simulink model "CTF"  (R2015a)
settings: Solver=ode15s  StartTime=0.0  StopTime=1e5  MaxStep=50  RelTol=1e-3
libraries: simCryogenics_lib x74, nesl_utility x45
settings Model: Creator=GM246266  LastModifiedBy=FB229602
settings SimscapeCC: SimscapeLogType=all

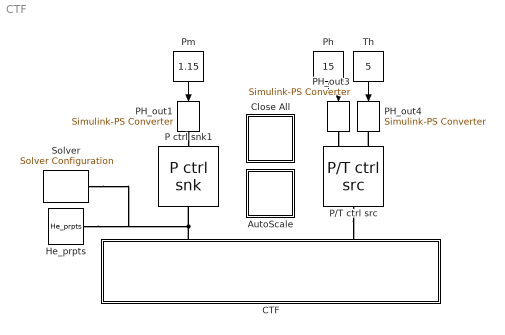
== system CTF ==
  AutoScale : Subsystem
      settings: OpenFcn=|
      | set(0, 'showhiddenhandles', 'on')
      | 
      | scope = findobj(0, 'Tag', 'SIMULINK_SIMSCOPE_FIGURE');
      | 
      | for i=1:length(scope)
      |   simscope('ScopeBar', 'ActionIcon', 'Find',     scope(i))
      | end
      | 
      | set(0, 'showhiddenhandles', 'off')
      mask Display: disp('Auto\nScale\nScope')
  CTF : Subsystem
  Close All : Subsystem
      settings: OpenFcn=|
      | set(0, 'showhiddenhandles', 'on')
      | scope = findobj(0, 'Tag','SIMULINK_SIMSCOPE_FIGURE');
      | close(scope)
      | set(0, 'showhiddenhandles', 'off')
      mask Display: disp('Close\nAll\nScope')
  He_prpts : simCryogenics_lib/Utilities/He_prpts  P_min=0.1 bar  T_min=3 K  T_max=8 K  P_max=20 bar  Mol=4.0026 * 10 ^ (- 3) kg/mol
  P ctrl snk1 : simCryogenics_lib/Sources_Sinks/P ctrl snk
  P/T ctrl src : simCryogenics_lib/Sources_Sinks/P//T ctrl src
  PH_out1 : nesl_utility/Simulink-PS Converter  PhysicalDomain=network_engine_domain  SubClassName=ps_input  LeftPortType=input  RightPortType=output  PseudoPeriodic=off  Frequencies=[]  NoiseDistribution=none  NoiseParameters=[]  Unit=bar  AffineConversion=off  InputFiltering=off  SimscapeFilterOrder=1  InputFilterTimeConstant=0.001  UdotUserProvided=1
  PH_out3 : nesl_utility/Simulink-PS Converter  PhysicalDomain=network_engine_domain  SubClassName=ps_input  LeftPortType=input  RightPortType=output  PseudoPeriodic=off  Frequencies=[]  NoiseDistribution=none  NoiseParameters=[]  Unit=bar  AffineConversion=off  InputFiltering=off  SimscapeFilterOrder=1  InputFilterTimeConstant=0.001  UdotUserProvided=1
  PH_out4 : nesl_utility/Simulink-PS Converter  PhysicalDomain=network_engine_domain  SubClassName=ps_input  LeftPortType=input  RightPortType=output  PseudoPeriodic=off  Frequencies=[]  NoiseDistribution=none  NoiseParameters=[]  Unit=K  AffineConversion=off  InputFiltering=off  SimscapeFilterOrder=1  InputFilterTimeConstant=0.001  UdotUserProvided=1
  Ph : Constant  Value=15
  Pm : Constant  Value=1.15
  Solver : nesl_utility/Solver Configuration  PhysicalDomain=network_engine_domain  SubClassName=solver  LeftPortType=input  RightPortType=generic  Accelerate=off  Tones=[]  Harmonics=[]  SimulateNoise=off  Profile=off  UseLocalSampling=off  EnableSwitchedLinearOptims=on  FrequencyDomain=off  UseCCode=off  RelTol=0.001  AbsTol=1e-06  MinStep=1e-09  ToWorkspace=off  RevertToSquareIcSolve=off  NumHomotopyIterations=100  DoDC=off  ResidualTolerance=1e-09  UseLocalSolver=off  LocalSolverChoice=NE_BACKWARD_EULER_ADVANCER  LocalSolverSampleTime=0.001  DoFixedCost=off  MaxNonlinIter=3  MaxModeIter=2  LinearAlgebra=Sparse  DelaysMemoryBudget=1024  AutomaticFiltering=on  FilteringTimeConstant=0.001
  Th : Constant  Value=5
  wires:
  Th/1 -> PH_out4/1
  Ph/1 -> PH_out3/1
  Pm/1 -> PH_out1/1
  connections:
  PH_out1/RConn1 -- P ctrl snk1/LConn1
  PH_out3/RConn1 -- P/T ctrl src/LConn1
  P/T ctrl src/LConn2 -- PH_out4/RConn1
  CTF/RConn1 -- Solver/RConn1 -- He_prpts/RConn1 -- P ctrl snk1/RConn1
  P/T ctrl src/RConn1 -- CTF/RConn2

== system CTF/AutoScale ==

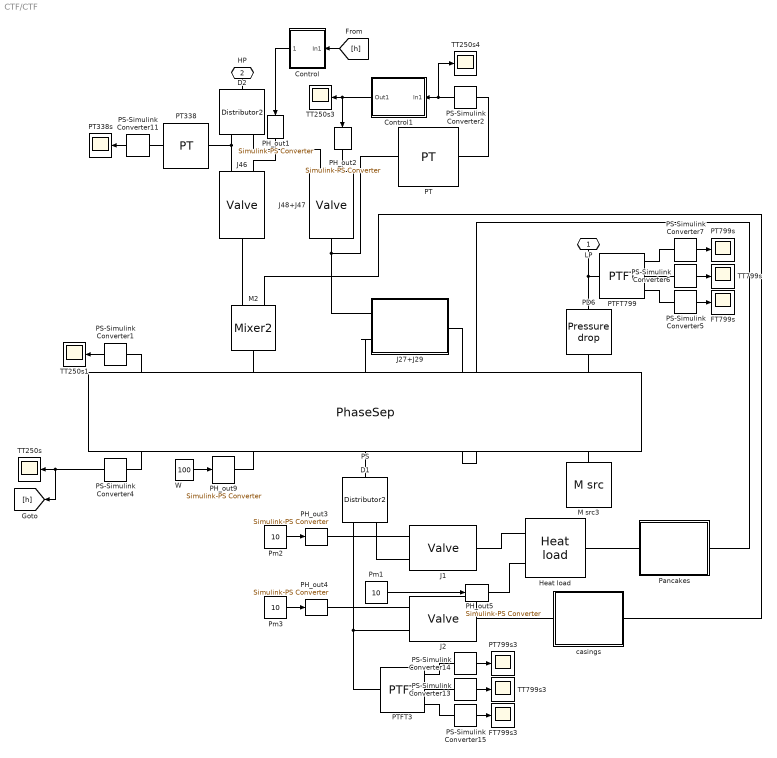
== system CTF/CTF ==
  Control : Subsystem
  Control1 : Subsystem
  D1 : simCryogenics_lib/Elements/Distributor2
  D2 : simCryogenics_lib/Elements/Distributor2
  FT799s : Scope
      settings: SaveName=FT799
  FT799s3 : Scope
      settings: SaveName=FT2
  Heat load : simCryogenics_lib/Utilities/Heat load
  J1 : simCryogenics_lib/Elements/Valve  CVmax=20  ControlInputMin=0  ControlInputMax=100  Xt=0.86  Rv=10  lin_v=0  lim_v=0  K=2.4e-5 m^1.50000*kg^0.50000/s/bar^0.50000  Cmd_specify=off  Cmd_priority=High  Cmd=0  gamma_specify=off  gamma_priority=High  gamma=0  rho_specify=off  rho_priority=High  rho=0 kg/m^3  Xc_specify=off  Xc_priority=High  Xc=0  X_specify=off  X_priority=High  X=0  Y_specify=off  Y_priority=High  Y=0  CV_specify=off  CV_priority=High  CV=0
  J2 : simCryogenics_lib/Elements/Valve  CVmax=25  ControlInputMin=0  ControlInputMax=100  Xt=0.86  Rv=10  lin_v=0  lim_v=0  K=2.4e-5 m^1.50000*kg^0.50000/s/bar^0.50000  Cmd_specify=off  Cmd_priority=High  Cmd=0  gamma_specify=off  gamma_priority=High  gamma=0  rho_specify=off  rho_priority=High  rho=0 kg/m^3  Xc_specify=off  Xc_priority=High  Xc=0  X_specify=off  X_priority=High  X=0  Y_specify=off  Y_priority=High  Y=0  CV_specify=off  CV_priority=High  CV=0
  J27+J29 : Subsystem
  J46 : simCryogenics_lib/Elements/Valve  CVmax=0.55  ControlInputMin=0  ControlInputMax=100  Xt=0.86  Rv=10  lin_v=0  lim_v=0  K=2.4e-5 m^1.50000*kg^0.50000/s/bar^0.50000  Cmd_specify=off  Cmd_priority=High  Cmd=0  gamma_specify=off  gamma_priority=High  gamma=0  rho_specify=off  rho_priority=High  rho=0 kg/m^3  Xc_specify=off  Xc_priority=High  Xc=0  X_specify=off  X_priority=High  X=0  Y_specify=off  Y_priority=High  Y=0  CV_specify=off  CV_priority=High  CV=0
  J48+J47 : simCryogenics_lib/Elements/Valve  CVmax=0.55  ControlInputMin=0  ControlInputMax=100  Xt=0.86  Rv=10  lin_v=0  lim_v=0  K=2.4e-5 m^1.50000*kg^0.50000/s/bar^0.50000  Cmd_specify=off  Cmd_priority=High  Cmd=0  gamma_specify=off  gamma_priority=High  gamma=0  rho_specify=off  rho_priority=High  rho=0 kg/m^3  Xc_specify=off  Xc_priority=High  Xc=0  X_specify=off  X_priority=High  X=0  Y_specify=off  Y_priority=High  Y=0  CV_specify=off  CV_priority=High  CV=0
  M src3 : simCryogenics_lib/Sources_Sinks/M src  M=0 kg/s
  M2 : simCryogenics_lib/Elements/Mixer2
  PD6 : simCryogenics_lib/Utilities/Pressure drop  K=1 s*bar/kg
  PH_out{1..4} (4 alike) : nesl_utility/Simulink-PS Converter  PhysicalDomain=network_engine_domain  SubClassName=ps_input  LeftPortType=input  RightPortType=output  PseudoPeriodic=off  Frequencies=[]  NoiseDistribution=none  NoiseParameters=[]  Unit=bar  AffineConversion=off  InputFiltering=off  SimscapeFilterOrder=1  InputFilterTimeConstant=0.001  UdotUserProvided=1
  PH_out5 : nesl_utility/Simulink-PS Converter  PhysicalDomain=network_engine_domain  SubClassName=ps_input  LeftPortType=input  RightPortType=output  PseudoPeriodic=off  Frequencies=[]  NoiseDistribution=none  NoiseParameters=[]  Unit=W  AffineConversion=off  InputFiltering=off  SimscapeFilterOrder=1  InputFilterTimeConstant=0.001  UdotUserProvided=1
  PH_out9 : nesl_utility/Simulink-PS Converter  PhysicalDomain=network_engine_domain  SubClassName=ps_input  LeftPortType=input  RightPortType=output  PseudoPeriodic=off  Frequencies=[]  NoiseDistribution=none  NoiseParameters=[]  Unit=1  AffineConversion=off  InputFiltering=off  SimscapeFilterOrder=1  InputFilterTimeConstant=0.001  UdotUserProvided=1
  PS : simCryogenics_lib/Elements/PhaseSep  Ideal1=1  DeltaT1=0.05 K  N1=1  h1=1 W/K  Ideal2=1  DeltaT2=0.05 K  N2=1  h2=1 W/K  hmax=1 m  S=1 m^2  P0=1.089 bar  h0=50
  PS-Simulink Converter{1..2,4..7,11,13..15} (10 alike) : nesl_utility/PS-Simulink Converter  PhysicalDomain=network_engine_domain  SubClassName=ps_output  LeftPortType=input  RightPortType=output  PseudoPeriodic=off  Frequencies=[]  Unit=1  AffineConversion=off
  PT : simCryogenics_lib/Sensors/PT
  PT338 : simCryogenics_lib/Sensors/PT
  PT338s : Scope
      settings: SaveName=PT1
  PT799s : Scope
      settings: SaveName=PT3
  PT799s3 : Scope
      settings: SaveName=PT4
  PTFT3 : simCryogenics_lib/Sensors/PTFT
  PTFT799 : simCryogenics_lib/Sensors/PTFT
  Pancakes : Subsystem
  Pm1 : Constant  Value=10
  Pm2 : Constant  Value=10
  Pm3 : Constant  Value=10
  TT250s{,1,3..4} (4 alike) : Scope
      TT250s settings: TimeRange=100000  YMin=49.99  YMax=50.08000000000001  SaveName=TT
      TT250s1 settings: SaveName=TT1
      TT250s3 settings: TimeRange=100000  YMin=49.99  YMax=50.08000000000001  SaveName=TT6
      TT250s4 settings: TimeRange=100000  YMin=1.8  YMax=3.1  SaveName=TT7
  TT799s : Scope
      settings: SaveName=TT799
  TT799s3 : Scope
      settings: SaveName=TT4
  W : Constant  Value=100
  casings : Subsystem
  LP : PMIOPort  Port=1  Side=Right
  HP : PMIOPort  Port=2  Side=Right
  wires:
  PS-Simulink Converter1/1 -> TT250s1/1
  W/1 -> PH_out9/1
  PS-Simulink Converter11/1 -> PT338s/1
  PS-Simulink Converter7/1 -> PT799s/1
  PS-Simulink Converter5/1 -> FT799s/1
  PS-Simulink Converter6/1 -> TT799s/1
  Control1/1(Out1) -> PH_out2/1, TT250s3/1
  Pm2/1 -> PH_out3/1
  Pm3/1 -> PH_out4/1
  PS-Simulink Converter14/1 -> PT799s3/1
  PS-Simulink Converter15/1 -> FT799s3/1
  PS-Simulink Converter13/1 -> TT799s3/1
  PS-Simulink Converter4/1 -> [h], TT250s/1
  Control/1(Out1) -> PH_out1/1
  PS-Simulink Converter2/1 -> TT250s4/1, Control1/1(In1)
  [h] -> Control/1(In1)
  Pm1/1 -> PH_out5/1
  connections:
  PT338/LConn1 -- J46/LConn2 -- D2/RConn2
  LP/RConn1 -- PD6/RConn1 -- PTFT799/LConn1
  M2/RConn1 -- PS/LConn4
  PS-Simulink Converter7/LConn1 -- PTFT799/RConn1
  PS-Simulink Converter1/LConn1 -- PS/LConn5
  M src3/RConn1 -- PS/RConn1
  PS-Simulink Converter5/LConn1 -- PTFT799/RConn3
  PS-Simulink Converter4/LConn1 -- PS/RConn5
  PS-Simulink Converter6/LConn1 -- PTFT799/RConn2
  PH_out9/RConn1 -- PS/RConn4
  PD6/LConn1 -- PS/LConn1
  PT338/RConn1 -- PS-Simulink Converter11/LConn1
  Pancakes/RConn1 -- PS/LConn2
  J27+J29/LConn2 -- PS/LConn3
  J27+J29/RConn1 -- PS/RConn2
  PT/LConn1 -- J48+J47/RConn1 -- J27+J29/LConn1
  J2/RConn1 -- casings/LConn1
  J46/RConn1 -- M2/LConn2
  D1/LConn1 -- PS/RConn3
  D1/RConn2 -- PTFT3/LConn1 -- J2/LConn2
  PH_out1/RConn1 -- J46/LConn1
  PH_out2/RConn1 -- J48+J47/LConn1
  PH_out3/RConn1 -- J1/LConn1
  J2/LConn1 -- PH_out4/RConn1
  HP/RConn1 -- D2/LConn1
  D2/RConn1 -- J48+J47/LConn2
  PS-Simulink Converter13/LConn1 -- PTFT3/RConn2
  PS-Simulink Converter15/LConn1 -- PTFT3/RConn3
  PS-Simulink Converter14/LConn1 -- PTFT3/RConn1
  D1/RConn1 -- J1/LConn2
  casings/RConn1 -- M2/LConn1
  PS-Simulink Converter2/LConn1 -- PT/RConn1
  PH_out5/RConn1 -- Heat load/LConn2
  J1/RConn1 -- Heat load/LConn1
  Heat load/RConn1 -- Pancakes/LConn1

== system CTF/Close All ==

== system CTF/CTF/Control ==
  In1 : Inport
  Bias : Bias  Bias=+60
  Gain : Gain  Gain=-1
  Out1 : Outport
  wires:
  Bias/1 -> Out1/1
  Gain/1 -> Bias/1
  In1/1 -> Gain/1

== system CTF/CTF/Control1 ==
  In1 : Inport
  Bias : Bias  Bias=-3
  Bias1 : Bias  Bias=10
  Gain : Gain  Gain=-10
  Out1 : Outport
  wires:
  Bias/1 -> Gain/1
  In1/1 -> Bias/1
  Gain/1 -> Bias1/1
  Bias1/1 -> Out1/1

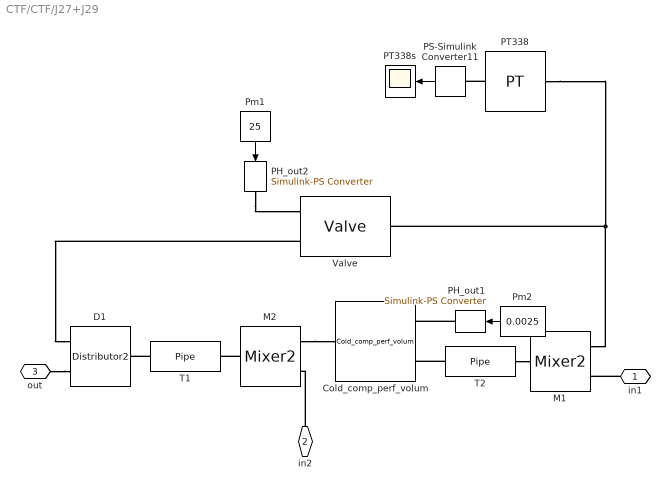
== system CTF/CTF/J27+J29 ==
  Cold_comp_perf_volum : simCryogenics_lib/Elements/Cold_comp_perf_volum  P0=1 bar  eta=0.8  Sin_specify=off  Sin_priority=High  Sin=0 kJ/kg  HoutIs_specify=off  HoutIs_priority=High  HoutIs=0 kJ/kg
  D1 : simCryogenics_lib/Elements/Distributor2
  M1 : simCryogenics_lib/Elements/Mixer2
  M2 : simCryogenics_lib/Elements/Mixer2
  PH_out1 : nesl_utility/Simulink-PS Converter  PhysicalDomain=network_engine_domain  SubClassName=ps_input  LeftPortType=input  RightPortType=output  PseudoPeriodic=off  Frequencies=[]  NoiseDistribution=none  NoiseParameters=[]  Unit=1  AffineConversion=off  InputFiltering=off  SimscapeFilterOrder=1  InputFilterTimeConstant=0.001  UdotUserProvided=1
  PH_out2 : nesl_utility/Simulink-PS Converter  PhysicalDomain=network_engine_domain  SubClassName=ps_input  LeftPortType=input  RightPortType=output  PseudoPeriodic=off  Frequencies=[]  NoiseDistribution=none  NoiseParameters=[]  Unit=bar  AffineConversion=off  InputFiltering=off  SimscapeFilterOrder=1  InputFilterTimeConstant=0.001  UdotUserProvided=1
  PS-Simulink Converter11 : nesl_utility/PS-Simulink Converter  PhysicalDomain=network_engine_domain  SubClassName=ps_output  LeftPortType=input  RightPortType=output  PseudoPeriodic=off  Frequencies=[]  Unit=1  AffineConversion=off
  PT338 : simCryogenics_lib/Sensors/PT
  PT338s : Scope
      settings: SaveName=PT5
  Pm1 : Constant  Value=25
  Pm2 : Constant  Value=0.0025
  T1 : simCryogenics_lib/Elements/Pipe  Vol=0.01 m^3  Ideal=0  P0=3 bar  T0=5 K
  T2 : simCryogenics_lib/Elements/Pipe  Vol=0.01 m^3  Ideal=0  P0=1 bar  T0=5 K
  Valve : simCryogenics_lib/Elements/Valve  CVmax=0.55  ControlInputMin=0  ControlInputMax=100  Xt=0.86  Rv=10  lin_v=0  lim_v=0  K=2.4e-5 m^1.50000*kg^0.50000/s/bar^0.50000  Cmd_specify=off  Cmd_priority=High  Cmd=0  gamma_specify=off  gamma_priority=High  gamma=0  rho_specify=off  rho_priority=High  rho=0 kg/m^3  Xc_specify=off  Xc_priority=High  Xc=0  X_specify=off  X_priority=High  X=0  Y_specify=off  Y_priority=High  Y=0  CV_specify=off  CV_priority=High  CV=0
  in1 : PMIOPort  Port=1  Side=Right
  in2 : PMIOPort  Port=2  Side=Left
  out : PMIOPort  Port=3  Side=Left
  wires:
  Pm1/1 -> PH_out2/1
  Pm2/1 -> PH_out1/1
  PS-Simulink Converter11/1 -> PT338s/1
  connections:
  T1/RConn1 -- D1/LConn1
  PH_out1/RConn1 -- Cold_comp_perf_volum/LConn2
  PH_out2/RConn1 -- Valve/LConn1
  Valve/LConn2 -- D1/RConn2
  out/RConn1 -- D1/RConn1
  in1/RConn1 -- M1/LConn1
  M1/LConn2 -- PT338/LConn1 -- Valve/RConn1
  T2/RConn1 -- Cold_comp_perf_volum/LConn1
  T2/LConn1 -- M1/RConn1
  M2/RConn1 -- T1/LConn1
  M2/LConn2 -- Cold_comp_perf_volum/RConn1
  in2/RConn1 -- M2/LConn1
  PT338/RConn1 -- PS-Simulink Converter11/LConn1

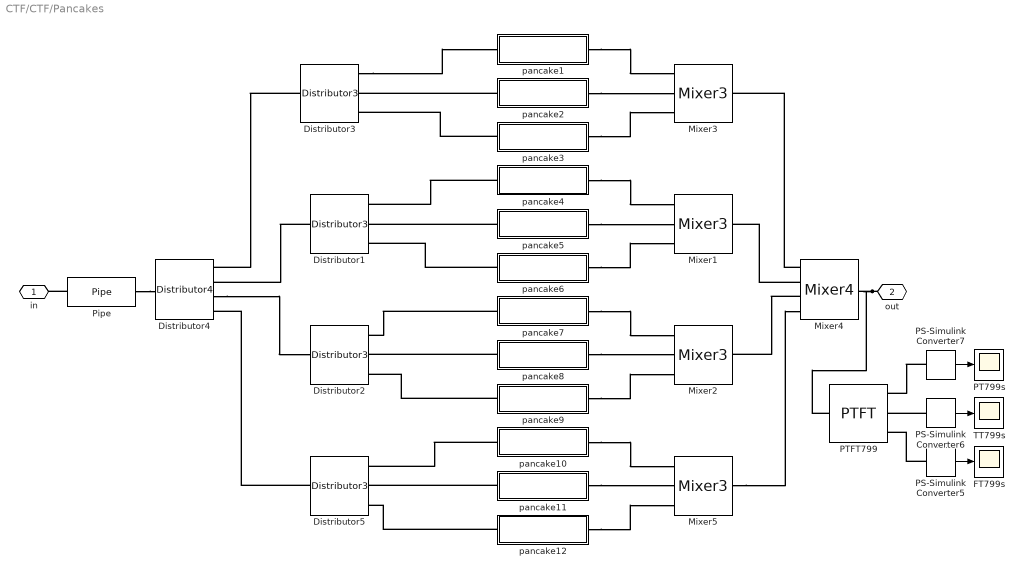
== system CTF/CTF/Pancakes ==
  Distributor{1..3,5} (4 alike) : simCryogenics_lib/Elements/Distributor3
  Distributor4 : simCryogenics_lib/Elements/Distributor4
  FT799s : Scope
      settings: SaveName=FT
  Mixer{1..3,5} (4 alike) : simCryogenics_lib/Elements/Mixer3
  Mixer4 : simCryogenics_lib/Elements/Mixer4
  PS-Simulink Converter5 : nesl_utility/PS-Simulink Converter  PhysicalDomain=network_engine_domain  SubClassName=ps_output  LeftPortType=input  RightPortType=output  PseudoPeriodic=off  Frequencies=[]  Unit=1  AffineConversion=off
  PS-Simulink Converter6 : nesl_utility/PS-Simulink Converter  PhysicalDomain=network_engine_domain  SubClassName=ps_output  LeftPortType=input  RightPortType=output  PseudoPeriodic=off  Frequencies=[]  Unit=1  AffineConversion=off
  PS-Simulink Converter7 : nesl_utility/PS-Simulink Converter  PhysicalDomain=network_engine_domain  SubClassName=ps_output  LeftPortType=input  RightPortType=output  PseudoPeriodic=off  Frequencies=[]  Unit=1  AffineConversion=off
  PT799s : Scope
      settings: TimeRange=1000  SaveName=PT
  PTFT799 : simCryogenics_lib/Sensors/PTFT
  Pipe : simCryogenics_lib/Elements/Pipe  Vol=1 m^3  Ideal=0  P0=2 bar  T0=5 K
  TT799s : Scope
      settings: YMin=5.00863  YMax=5.00863  SaveName=TT2
  pancake1 : Subsystem
  pancake10 : Subsystem
  pancake11 : Subsystem
  pancake12 : Subsystem
  pancake2 : Subsystem
  pancake3 : Subsystem
  pancake4 : Subsystem
  pancake5 : Subsystem
  pancake6 : Subsystem
  pancake7 : Subsystem
  pancake8 : Subsystem
  pancake9 : Subsystem
  in : PMIOPort  Port=1  Side=Left
  out : PMIOPort  Port=2  Side=Right
  wires:
  PS-Simulink Converter7/1 -> PT799s/1
  PS-Simulink Converter5/1 -> FT799s/1
  PS-Simulink Converter6/1 -> TT799s/1
  connections:
  PS-Simulink Converter5/LConn1 -- PTFT799/RConn3
  PS-Simulink Converter7/LConn1 -- PTFT799/RConn1
  PS-Simulink Converter6/LConn1 -- PTFT799/RConn2
  Pipe/LConn1 -- in/RConn1
  Distributor3/LConn1 -- Distributor4/RConn1
  Distributor1/LConn1 -- Distributor4/RConn2
  Distributor4/RConn3 -- Distributor2/LConn1
  Distributor5/LConn1 -- Distributor4/RConn4
  Distributor3/RConn1 -- pancake1/LConn1
  pancake2/LConn1 -- Distributor3/RConn2
  pancake3/LConn1 -- Distributor3/RConn3
  pancake4/LConn1 -- Distributor1/RConn1
  pancake5/LConn1 -- Distributor1/RConn2
  pancake6/LConn1 -- Distributor1/RConn3
  pancake7/LConn1 -- Distributor2/RConn1
  pancake8/LConn1 -- Distributor2/RConn2
  pancake9/LConn1 -- Distributor2/RConn3
  pancake11/LConn1 -- Distributor5/RConn2
  pancake10/LConn1 -- Distributor5/RConn1
  pancake12/LConn1 -- Distributor5/RConn3
  pancake2/RConn1 -- Mixer3/LConn2
  pancake1/RConn1 -- Mixer3/LConn1
  pancake3/RConn1 -- Mixer3/LConn3
  pancake4/RConn1 -- Mixer1/LConn1
  pancake5/RConn1 -- Mixer1/LConn2
  pancake6/RConn1 -- Mixer1/LConn3
  pancake7/RConn1 -- Mixer2/LConn1
  pancake8/RConn1 -- Mixer2/LConn2
  pancake9/RConn1 -- Mixer2/LConn3
  pancake10/RConn1 -- Mixer5/LConn1
  pancake11/RConn1 -- Mixer5/LConn2
  pancake12/RConn1 -- Mixer5/LConn3
  Mixer4/LConn2 -- Mixer1/RConn1
  Mixer4/LConn1 -- Mixer3/RConn1
  Mixer4/LConn3 -- Mixer2/RConn1
  Mixer5/RConn1 -- Mixer4/LConn4
  Mixer4/RConn1 -- out/RConn1 -- PTFT799/LConn1
  Pipe/RConn1 -- Distributor4/LConn1

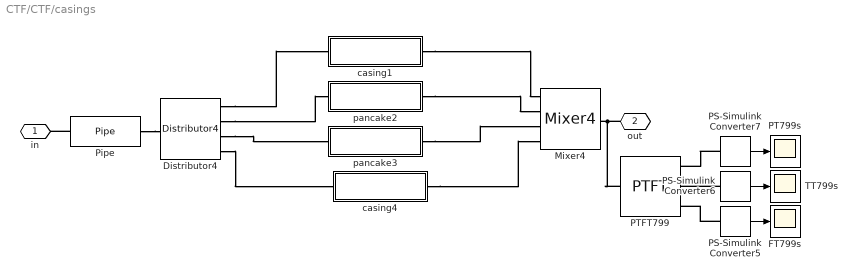
== system CTF/CTF/casings ==
  Distributor4 : simCryogenics_lib/Elements/Distributor4
  FT799s : Scope
      settings: SaveName=FT1
  Mixer4 : simCryogenics_lib/Elements/Mixer4
  PS-Simulink Converter5 : nesl_utility/PS-Simulink Converter  PhysicalDomain=network_engine_domain  SubClassName=ps_output  LeftPortType=input  RightPortType=output  PseudoPeriodic=off  Frequencies=[]  Unit=1  AffineConversion=off
  PS-Simulink Converter6 : nesl_utility/PS-Simulink Converter  PhysicalDomain=network_engine_domain  SubClassName=ps_output  LeftPortType=input  RightPortType=output  PseudoPeriodic=off  Frequencies=[]  Unit=1  AffineConversion=off
  PS-Simulink Converter7 : nesl_utility/PS-Simulink Converter  PhysicalDomain=network_engine_domain  SubClassName=ps_output  LeftPortType=input  RightPortType=output  PseudoPeriodic=off  Frequencies=[]  Unit=1  AffineConversion=off
  PT799s : Scope
      settings: SaveName=PT2
  PTFT799 : simCryogenics_lib/Sensors/PTFT
  Pipe : simCryogenics_lib/Elements/Pipe  Vol=1 m^3  Ideal=0  P0=2 bar  T0=5 K
  TT799s : Scope
      settings: SaveName=TT5
  casing1 : Subsystem
  casing4 : Subsystem
  pancake2 : Subsystem
  pancake3 : Subsystem
  in : PMIOPort  Port=1  Side=Left
  out : PMIOPort  Port=2  Side=Right
  wires:
  PS-Simulink Converter7/1 -> PT799s/1
  PS-Simulink Converter5/1 -> FT799s/1
  PS-Simulink Converter6/1 -> TT799s/1
  connections:
  Pipe/RConn1 -- Distributor4/LConn1
  out/RConn1 -- PTFT799/LConn1 -- Mixer4/RConn1
  casing4/RConn1 -- Mixer4/LConn4
  pancake3/RConn1 -- Mixer4/LConn3
  casing1/RConn1 -- Mixer4/LConn1
  pancake2/RConn1 -- Mixer4/LConn2
  Distributor4/RConn4 -- casing4/LConn1
  Distributor4/RConn3 -- pancake3/LConn1
  Distributor4/RConn2 -- pancake2/LConn1
  Distributor4/RConn1 -- casing1/LConn1
  Pipe/LConn1 -- in/RConn1
  PS-Simulink Converter5/LConn1 -- PTFT799/RConn3
  PS-Simulink Converter7/LConn1 -- PTFT799/RConn1
  PS-Simulink Converter6/LConn1 -- PTFT799/RConn2

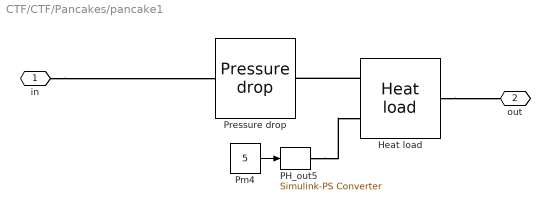
== system CTF/CTF/Pancakes/pancake1 ==
  Heat load : simCryogenics_lib/Utilities/Heat load
  PH_out5 : nesl_utility/Simulink-PS Converter  PhysicalDomain=network_engine_domain  SubClassName=ps_input  LeftPortType=input  RightPortType=output  PseudoPeriodic=off  Frequencies=[]  NoiseDistribution=none  NoiseParameters=[]  Unit=W  AffineConversion=off  InputFiltering=off  SimscapeFilterOrder=1  InputFilterTimeConstant=0.001  UdotUserProvided=1
  Pm4 : Constant  Value=5
  Pressure drop : simCryogenics_lib/Utilities/Pressure drop  K=1/0.0025 s*bar/kg
  in : PMIOPort  Port=1  Side=Left
  out : PMIOPort  Port=2  Side=Right
  wires:
  Pm4/1 -> PH_out5/1
  connections:
  PH_out5/RConn1 -- Heat load/LConn2
  Heat load/RConn1 -- out/RConn1
  in/RConn1 -- Pressure drop/LConn1
  Heat load/LConn1 -- Pressure drop/RConn1

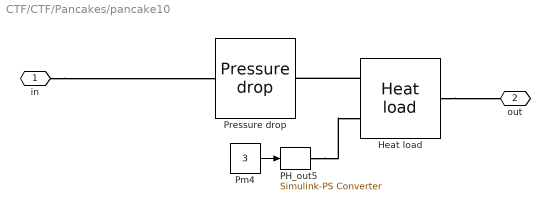
== system CTF/CTF/Pancakes/pancake10 ==
  Heat load : simCryogenics_lib/Utilities/Heat load
  PH_out5 : nesl_utility/Simulink-PS Converter  PhysicalDomain=network_engine_domain  SubClassName=ps_input  LeftPortType=input  RightPortType=output  PseudoPeriodic=off  Frequencies=[]  NoiseDistribution=none  NoiseParameters=[]  Unit=W  AffineConversion=off  InputFiltering=off  SimscapeFilterOrder=1  InputFilterTimeConstant=0.001  UdotUserProvided=1
  Pm4 : Constant  Value=3
  Pressure drop : simCryogenics_lib/Utilities/Pressure drop  K=1/0.0025 s*bar/kg
  in : PMIOPort  Port=1  Side=Left
  out : PMIOPort  Port=2  Side=Right
  wires:
  Pm4/1 -> PH_out5/1
  connections:
  Heat load/LConn1 -- Pressure drop/RConn1
  in/RConn1 -- Pressure drop/LConn1
  Heat load/RConn1 -- out/RConn1
  PH_out5/RConn1 -- Heat load/LConn2

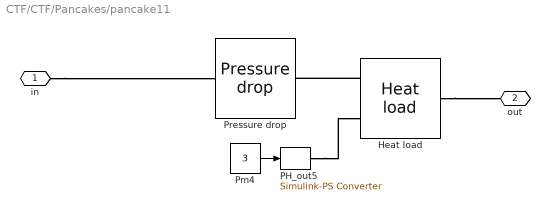
== system CTF/CTF/Pancakes/pancake11 ==
  Heat load : simCryogenics_lib/Utilities/Heat load
  PH_out5 : nesl_utility/Simulink-PS Converter  PhysicalDomain=network_engine_domain  SubClassName=ps_input  LeftPortType=input  RightPortType=output  PseudoPeriodic=off  Frequencies=[]  NoiseDistribution=none  NoiseParameters=[]  Unit=W  AffineConversion=off  InputFiltering=off  SimscapeFilterOrder=1  InputFilterTimeConstant=0.001  UdotUserProvided=1
  Pm4 : Constant  Value=3
  Pressure drop : simCryogenics_lib/Utilities/Pressure drop  K=1/0.0025 s*bar/kg
  in : PMIOPort  Port=1  Side=Left
  out : PMIOPort  Port=2  Side=Right
  wires:
  Pm4/1 -> PH_out5/1
  connections:
  PH_out5/RConn1 -- Heat load/LConn2
  Heat load/RConn1 -- out/RConn1
  in/RConn1 -- Pressure drop/LConn1
  Heat load/LConn1 -- Pressure drop/RConn1

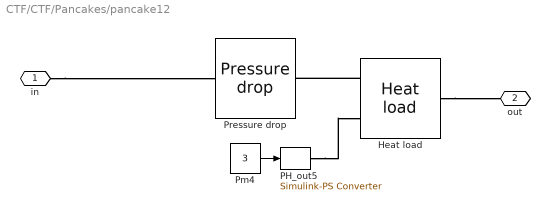
== system CTF/CTF/Pancakes/pancake12 ==
  Heat load : simCryogenics_lib/Utilities/Heat load
  PH_out5 : nesl_utility/Simulink-PS Converter  PhysicalDomain=network_engine_domain  SubClassName=ps_input  LeftPortType=input  RightPortType=output  PseudoPeriodic=off  Frequencies=[]  NoiseDistribution=none  NoiseParameters=[]  Unit=W  AffineConversion=off  InputFiltering=off  SimscapeFilterOrder=1  InputFilterTimeConstant=0.001  UdotUserProvided=1
  Pm4 : Constant  Value=3
  Pressure drop : simCryogenics_lib/Utilities/Pressure drop  K=1/0.0025 s*bar/kg
  in : PMIOPort  Port=1  Side=Left
  out : PMIOPort  Port=2  Side=Right
  wires:
  Pm4/1 -> PH_out5/1
  connections:
  Heat load/LConn1 -- Pressure drop/RConn1
  in/RConn1 -- Pressure drop/LConn1
  Heat load/RConn1 -- out/RConn1
  PH_out5/RConn1 -- Heat load/LConn2

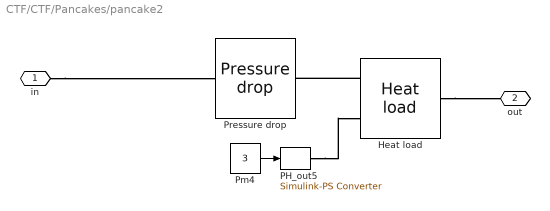
== system CTF/CTF/Pancakes/pancake2 ==
  Heat load : simCryogenics_lib/Utilities/Heat load
  PH_out5 : nesl_utility/Simulink-PS Converter  PhysicalDomain=network_engine_domain  SubClassName=ps_input  LeftPortType=input  RightPortType=output  PseudoPeriodic=off  Frequencies=[]  NoiseDistribution=none  NoiseParameters=[]  Unit=W  AffineConversion=off  InputFiltering=off  SimscapeFilterOrder=1  InputFilterTimeConstant=0.001  UdotUserProvided=1
  Pm4 : Constant  Value=3
  Pressure drop : simCryogenics_lib/Utilities/Pressure drop  K=1/0.0025 s*bar/kg
  in : PMIOPort  Port=1  Side=Left
  out : PMIOPort  Port=2  Side=Right
  wires:
  Pm4/1 -> PH_out5/1
  connections:
  Heat load/LConn1 -- Pressure drop/RConn1
  in/RConn1 -- Pressure drop/LConn1
  Heat load/RConn1 -- out/RConn1
  PH_out5/RConn1 -- Heat load/LConn2

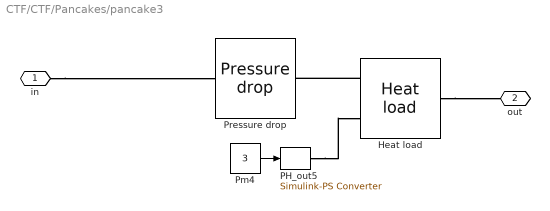
== system CTF/CTF/Pancakes/pancake3 ==
  Heat load : simCryogenics_lib/Utilities/Heat load
  PH_out5 : nesl_utility/Simulink-PS Converter  PhysicalDomain=network_engine_domain  SubClassName=ps_input  LeftPortType=input  RightPortType=output  PseudoPeriodic=off  Frequencies=[]  NoiseDistribution=none  NoiseParameters=[]  Unit=W  AffineConversion=off  InputFiltering=off  SimscapeFilterOrder=1  InputFilterTimeConstant=0.001  UdotUserProvided=1
  Pm4 : Constant  Value=3
  Pressure drop : simCryogenics_lib/Utilities/Pressure drop  K=1/0.0025 s*bar/kg
  in : PMIOPort  Port=1  Side=Left
  out : PMIOPort  Port=2  Side=Right
  wires:
  Pm4/1 -> PH_out5/1
  connections:
  PH_out5/RConn1 -- Heat load/LConn2
  Heat load/RConn1 -- out/RConn1
  in/RConn1 -- Pressure drop/LConn1
  Heat load/LConn1 -- Pressure drop/RConn1

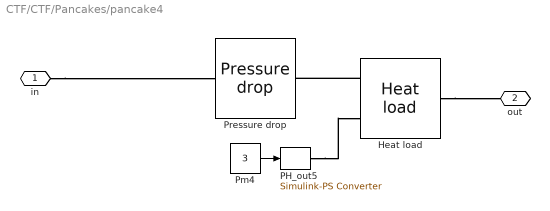
== system CTF/CTF/Pancakes/pancake4 ==
  Heat load : simCryogenics_lib/Utilities/Heat load
  PH_out5 : nesl_utility/Simulink-PS Converter  PhysicalDomain=network_engine_domain  SubClassName=ps_input  LeftPortType=input  RightPortType=output  PseudoPeriodic=off  Frequencies=[]  NoiseDistribution=none  NoiseParameters=[]  Unit=W  AffineConversion=off  InputFiltering=off  SimscapeFilterOrder=1  InputFilterTimeConstant=0.001  UdotUserProvided=1
  Pm4 : Constant  Value=3
  Pressure drop : simCryogenics_lib/Utilities/Pressure drop  K=1/0.0025 s*bar/kg
  in : PMIOPort  Port=1  Side=Left
  out : PMIOPort  Port=2  Side=Right
  wires:
  Pm4/1 -> PH_out5/1
  connections:
  Heat load/LConn1 -- Pressure drop/RConn1
  in/RConn1 -- Pressure drop/LConn1
  Heat load/RConn1 -- out/RConn1
  PH_out5/RConn1 -- Heat load/LConn2

== system CTF/CTF/Pancakes/pancake5 ==
  Heat load : simCryogenics_lib/Utilities/Heat load
  PH_out5 : nesl_utility/Simulink-PS Converter  PhysicalDomain=network_engine_domain  SubClassName=ps_input  LeftPortType=input  RightPortType=output  PseudoPeriodic=off  Frequencies=[]  NoiseDistribution=none  NoiseParameters=[]  Unit=W  AffineConversion=off  InputFiltering=off  SimscapeFilterOrder=1  InputFilterTimeConstant=0.001  UdotUserProvided=1
  Pm4 : Constant  Value=3
  Pressure drop : simCryogenics_lib/Utilities/Pressure drop  K=1/0.0025 s*bar/kg
  in : PMIOPort  Port=1  Side=Left
  out : PMIOPort  Port=2  Side=Right
  wires:
  Pm4/1 -> PH_out5/1
  connections:
  PH_out5/RConn1 -- Heat load/LConn2
  Heat load/RConn1 -- out/RConn1
  in/RConn1 -- Pressure drop/LConn1
  Heat load/LConn1 -- Pressure drop/RConn1

== system CTF/CTF/Pancakes/pancake6 ==
  Heat load : simCryogenics_lib/Utilities/Heat load
  PH_out5 : nesl_utility/Simulink-PS Converter  PhysicalDomain=network_engine_domain  SubClassName=ps_input  LeftPortType=input  RightPortType=output  PseudoPeriodic=off  Frequencies=[]  NoiseDistribution=none  NoiseParameters=[]  Unit=W  AffineConversion=off  InputFiltering=off  SimscapeFilterOrder=1  InputFilterTimeConstant=0.001  UdotUserProvided=1
  Pm4 : Constant  Value=3
  Pressure drop : simCryogenics_lib/Utilities/Pressure drop  K=1/0.0025 s*bar/kg
  in : PMIOPort  Port=1  Side=Left
  out : PMIOPort  Port=2  Side=Right
  wires:
  Pm4/1 -> PH_out5/1
  connections:
  Heat load/LConn1 -- Pressure drop/RConn1
  in/RConn1 -- Pressure drop/LConn1
  Heat load/RConn1 -- out/RConn1
  PH_out5/RConn1 -- Heat load/LConn2

== system CTF/CTF/Pancakes/pancake7 ==
  Heat load : simCryogenics_lib/Utilities/Heat load
  PH_out5 : nesl_utility/Simulink-PS Converter  PhysicalDomain=network_engine_domain  SubClassName=ps_input  LeftPortType=input  RightPortType=output  PseudoPeriodic=off  Frequencies=[]  NoiseDistribution=none  NoiseParameters=[]  Unit=W  AffineConversion=off  InputFiltering=off  SimscapeFilterOrder=1  InputFilterTimeConstant=0.001  UdotUserProvided=1
  Pm4 : Constant  Value=3
  Pressure drop : simCryogenics_lib/Utilities/Pressure drop  K=1/0.0025 s*bar/kg
  in : PMIOPort  Port=1  Side=Left
  out : PMIOPort  Port=2  Side=Right
  wires:
  Pm4/1 -> PH_out5/1
  connections:
  PH_out5/RConn1 -- Heat load/LConn2
  Heat load/RConn1 -- out/RConn1
  in/RConn1 -- Pressure drop/LConn1
  Heat load/LConn1 -- Pressure drop/RConn1

== system CTF/CTF/Pancakes/pancake8 ==
  Heat load : simCryogenics_lib/Utilities/Heat load
  PH_out5 : nesl_utility/Simulink-PS Converter  PhysicalDomain=network_engine_domain  SubClassName=ps_input  LeftPortType=input  RightPortType=output  PseudoPeriodic=off  Frequencies=[]  NoiseDistribution=none  NoiseParameters=[]  Unit=W  AffineConversion=off  InputFiltering=off  SimscapeFilterOrder=1  InputFilterTimeConstant=0.001  UdotUserProvided=1
  Pm4 : Constant  Value=3
  Pressure drop : simCryogenics_lib/Utilities/Pressure drop  K=1/0.0025 s*bar/kg
  in : PMIOPort  Port=1  Side=Left
  out : PMIOPort  Port=2  Side=Right
  wires:
  Pm4/1 -> PH_out5/1
  connections:
  Heat load/LConn1 -- Pressure drop/RConn1
  in/RConn1 -- Pressure drop/LConn1
  Heat load/RConn1 -- out/RConn1
  PH_out5/RConn1 -- Heat load/LConn2

== system CTF/CTF/Pancakes/pancake9 ==
  Heat load : simCryogenics_lib/Utilities/Heat load
  PH_out5 : nesl_utility/Simulink-PS Converter  PhysicalDomain=network_engine_domain  SubClassName=ps_input  LeftPortType=input  RightPortType=output  PseudoPeriodic=off  Frequencies=[]  NoiseDistribution=none  NoiseParameters=[]  Unit=W  AffineConversion=off  InputFiltering=off  SimscapeFilterOrder=1  InputFilterTimeConstant=0.001  UdotUserProvided=1
  Pm4 : Constant  Value=3
  Pressure drop : simCryogenics_lib/Utilities/Pressure drop  K=1/0.0025 s*bar/kg
  in : PMIOPort  Port=1  Side=Left
  out : PMIOPort  Port=2  Side=Right
  wires:
  Pm4/1 -> PH_out5/1
  connections:
  PH_out5/RConn1 -- Heat load/LConn2
  Heat load/RConn1 -- out/RConn1
  in/RConn1 -- Pressure drop/LConn1
  Heat load/LConn1 -- Pressure drop/RConn1

== system CTF/CTF/casings/casing1 ==
  Heat load : simCryogenics_lib/Utilities/Heat load
  PH_out5 : nesl_utility/Simulink-PS Converter  PhysicalDomain=network_engine_domain  SubClassName=ps_input  LeftPortType=input  RightPortType=output  PseudoPeriodic=off  Frequencies=[]  NoiseDistribution=none  NoiseParameters=[]  Unit=W  AffineConversion=off  InputFiltering=off  SimscapeFilterOrder=1  InputFilterTimeConstant=0.001  UdotUserProvided=1
  Pm4 : Constant  Value=5
  Pressure drop : simCryogenics_lib/Utilities/Pressure drop  K=1/0.0025 s*bar/kg
  in : PMIOPort  Port=1  Side=Left
  out : PMIOPort  Port=2  Side=Right
  wires:
  Pm4/1 -> PH_out5/1
  connections:
  Heat load/LConn1 -- Pressure drop/RConn1
  in/RConn1 -- Pressure drop/LConn1
  Heat load/RConn1 -- out/RConn1
  PH_out5/RConn1 -- Heat load/LConn2

== system CTF/CTF/casings/casing4 ==
  Heat load : simCryogenics_lib/Utilities/Heat load
  PH_out5 : nesl_utility/Simulink-PS Converter  PhysicalDomain=network_engine_domain  SubClassName=ps_input  LeftPortType=input  RightPortType=output  PseudoPeriodic=off  Frequencies=[]  NoiseDistribution=none  NoiseParameters=[]  Unit=W  AffineConversion=off  InputFiltering=off  SimscapeFilterOrder=1  InputFilterTimeConstant=0.001  UdotUserProvided=1
  Pm4 : Constant  Value=3
  Pressure drop : simCryogenics_lib/Utilities/Pressure drop  K=1/0.0025 s*bar/kg
  in : PMIOPort  Port=1  Side=Left
  out : PMIOPort  Port=2  Side=Right
  wires:
  Pm4/1 -> PH_out5/1
  connections:
  PH_out5/RConn1 -- Heat load/LConn2
  Heat load/RConn1 -- out/RConn1
  in/RConn1 -- Pressure drop/LConn1
  Heat load/LConn1 -- Pressure drop/RConn1

== system CTF/CTF/casings/pancake2 ==
  Heat load : simCryogenics_lib/Utilities/Heat load
  PH_out5 : nesl_utility/Simulink-PS Converter  PhysicalDomain=network_engine_domain  SubClassName=ps_input  LeftPortType=input  RightPortType=output  PseudoPeriodic=off  Frequencies=[]  NoiseDistribution=none  NoiseParameters=[]  Unit=W  AffineConversion=off  InputFiltering=off  SimscapeFilterOrder=1  InputFilterTimeConstant=0.001  UdotUserProvided=1
  Pm4 : Constant  Value=3
  Pressure drop : simCryogenics_lib/Utilities/Pressure drop  K=1/0.0025 s*bar/kg
  in : PMIOPort  Port=1  Side=Left
  out : PMIOPort  Port=2  Side=Right
  wires:
  Pm4/1 -> PH_out5/1
  connections:
  PH_out5/RConn1 -- Heat load/LConn2
  Heat load/RConn1 -- out/RConn1
  in/RConn1 -- Pressure drop/LConn1
  Heat load/LConn1 -- Pressure drop/RConn1

== system CTF/CTF/casings/pancake3 ==
  Heat load : simCryogenics_lib/Utilities/Heat load
  PH_out5 : nesl_utility/Simulink-PS Converter  PhysicalDomain=network_engine_domain  SubClassName=ps_input  LeftPortType=input  RightPortType=output  PseudoPeriodic=off  Frequencies=[]  NoiseDistribution=none  NoiseParameters=[]  Unit=W  AffineConversion=off  InputFiltering=off  SimscapeFilterOrder=1  InputFilterTimeConstant=0.001  UdotUserProvided=1
  Pm4 : Constant  Value=3
  Pressure drop : simCryogenics_lib/Utilities/Pressure drop  K=1/0.0025 s*bar/kg
  in : PMIOPort  Port=1  Side=Left
  out : PMIOPort  Port=2  Side=Right
  wires:
  Pm4/1 -> PH_out5/1
  connections:
  Heat load/LConn1 -- Pressure drop/RConn1
  in/RConn1 -- Pressure drop/LConn1
  Heat load/RConn1 -- out/RConn1
  PH_out5/RConn1 -- Heat load/LConn2
